simulink model "Sistema_completo"  (R2020b)
settings: Solver=FixedStepAuto  StartTime=0.0  StopTime=inf  FixedStep=0.01  RelTol=1e-3  EnableMultiTasking=on
values from neighbouring files (symbols this model uses):
  a_c_max = 1    [Parametros_y_Simulacion.m]
  a_i_max = 1    [Parametros_y_Simulacion.m]
  b_cx = 1000.0    (= 1000)    [Parametros_y_Simulacion.m]
  b_cy = 500.0    (= 500)    [Parametros_y_Simulacion.m]
  b_eqc = b_eq * r_t^2 / R_r^2    (= 27000)    [Parametros_y_Simulacion.m]
  b_eqi = b_eq2 * r_ti^2 / R_d^2    (= 28800)    [Parametros_y_Simulacion.m]
  b_w = 30000.0    (= 30000)    [Parametros_y_Simulacion.m]
  g = 9.81    [Parametros_y_Simulacion.m]
  H_colmn = [34,34, 19,19, 35,30, 35,30, 23]    [Parametros_y_Simulacion.m]
  H_contenedor = 2.5    [Parametros_y_Simulacion.m]
  H_seguridad = 5    [Parametros_y_Simulacion.m]
  K_cy = 1.3e6    (= 1300000)    [Parametros_y_Simulacion.m]
  K_w = 1800000.0    (= 1800000)    [Parametros_y_Simulacion.m]
  L_colmn = [5,10,15, 20,25, 30,35, 40,45]    [Parametros_y_Simulacion.m]
  l_t0 = y_t0 - H_contenedor - H_seguridad -(m_spreader * g) / K_w    (= 37.41825)    [Parametros_y_Simulacion.m]
  m_carga = 48000.0    (= 48000)    [Parametros_y_Simulacion.m]
  m_eqc = m_c + (J_r + J_m * r_t^2) / (R_r^2)    (= 59008)    [Parametros_y_Simulacion.m]
  m_eqi = (J_d + J_mi * r_ti^2) / R_d^2    (= 48014.2222222)    [Parametros_y_Simulacion.m]
  m_spreader = 15000.0    (= 15000)    [Parametros_y_Simulacion.m]
  omega_c_mod = 1000    [Parametros_y_Simulacion.m]
  omega_i_mod = 1000    [Parametros_y_Simulacion.m]
  R_d = 0.75    [Parametros_y_Simulacion.m]
  R_r = 0.5    [Parametros_y_Simulacion.m]
  r_t = 15.0    (= 15)    [Parametros_y_Simulacion.m]
  r_ti = 30.0    (= 30)    [Parametros_y_Simulacion.m]
  v_c_max = 4    [Parametros_y_Simulacion.m]
  x_t0 = -20    [Parametros_y_Simulacion.m]
  y_t0 = 45    [Parametros_y_Simulacion.m]
undefined symbols (not defined in the file or in its folder): B_ac, B_ai, H, K_db, K_pb, K_sac, K_sai, K_siac, K_siai, L, lh
libraries: aerolibanimutils x1
settings Model: Creator=Facundo  LastModifiedBy=tinsu
settings DataIOCC: LimitDataPoints=on  ReturnWorkspaceOutputs=off
settings OptimizationCC: ZeroExternalMemoryAtStartup=off  ZeroInternalMemoryAtStartup=off  LifeSpan=inf
settings DebuggingCC: SFUnexpectedBacktrackingDiag=warning  SFNoUnconditionalDefaultTransitionDiag=warning  SFExecutionAtInitializationDiag=none  ArithmeticOperatorsInVariantConditions=warning
settings HardwareCC: ProdBitPerSizeT=32  ProdBitPerPtrDiffT=32  ProdWordSize=32  ProdHWDeviceType=Specified
settings ModelReferenceCC: PropagateSignalLabelsOutOfModel=off
settings SFSimCC: SimUseLocalCustomCode=off  CustomCodeUndefinedFunction=UseInterfaceOnly  SimTargetLang=C++
settings RTWCC: RTWUseLocalCustomCode=off  TargetLang=C++
settings CodeAppCC: StateflowObjectComments=on
settings GRTTargetCC: TargetLangStandard=C89/C90 (ANSI)  CodeInterfacePackaging=C++ class  RTWCAPISignals=on
settings ConfigComp: CovMetricSettings=dw  CovSaveCumulativeToWorkspaceVar=on  CovSaveSingleToWorkspaceVar=on  CovExternalEMLEnable=off

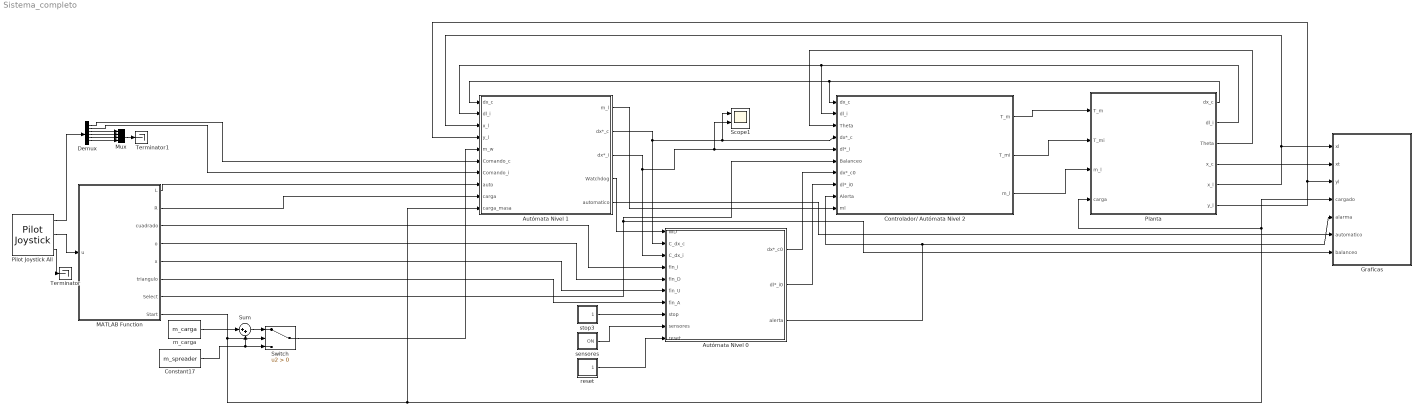
== system Sistema_completo ==
  " Planta" : Subsystem
  Autómata Nivel 0 : Subsystem
  Autómata Nivel 1 : Subsystem
  Constant17 : Constant  Value=m_spreader
  Controlador/ Autómata Nivel 2 : Subsystem
  Demux : Demux  Outputs=6
  Graficas : Stateflow chart  TreatAsAtomicUnit=on
  MATLAB Function : MATLAB Function  TreatAsAtomicUnit=on
  Mux : Mux
  Pilot Joystick All : aerolibanimutils/Pilot Joystick  JoystickID=Joystick1  OutputConfiguration=AllOutputs  SampleTime=0.01
  Scope1 : Scope  NumInputPorts=2
  Sum : Sum  Inputs=|++
  Switch : Switch  Criteria=u2 > Threshold
  Terminator : Terminator
  Terminator1 : Terminator
  m_carga : Constant  Value=m_carga
  reset : Subsystem
      settings: OpenFcn=|
      | blockname1=[gcb '/ControlValue/'];
      | blockname2=[gcb '/'];
      | 
      | h1=get_param(blockname1,'handle');
      | h2=get_param(blockname2,'handle');
      | ONOFF=str2num(get_param(h1,'Value'));
      | 
      | if ONOFF== 1
      |     %Turn off
      |     set_param(h1,'Value','-1')
      |     set_param(h2,'BackgroundColor','blue')
      |     set_param([gcb '/ON'],'Name','OFF')
      | else
      |     %Turn on
      |     set_param(h1,'Value','1')
      |     set_param(h2,'BackgroundColor','red')
      |     set_param([gcb '/OFF'],'Name','ON')
      | end
  sensores : Subsystem
      settings: OpenFcn=|
      | blockname1=[gcb '/ControlValue/'];
      | blockname2=[gcb '/'];
      | 
      | h1=get_param(blockname1,'handle');
      | h2=get_param(blockname2,'handle');
      | ONOFF=str2num(get_param(h1,'Value'));
      | 
      | if ONOFF== 1
      |     %Turn off
      |     set_param(h1,'Value','-1')
      |     set_param(h2,'BackgroundColor','blue')
      |     set_param([gcb '/ON'],'Name','OFF')
      | else
      |     %Turn on
      |     set_param(h1,'Value','1')
      |     set_param(h2,'BackgroundColor','red')
      |     set_param([gcb '/OFF'],'Name','ON')
      | end
  stop3 : Subsystem
      settings: OpenFcn=|
      | blockname1=[gcb '/ControlValue/'];
      | blockname2=[gcb '/'];
      | 
      | h1=get_param(blockname1,'handle');
      | h2=get_param(blockname2,'handle');
      | ONOFF=str2num(get_param(h1,'Value'));
      | 
      | if ONOFF== 1
      |     %Turn off
      |     set_param(h1,'Value','-1')
      |     set_param(h2,'BackgroundColor','blue')
      |     set_param([gcb '/ON'],'Name','OFF')
      | else
      |     %Turn on
      |     set_param(h1,'Value','1')
      |     set_param(h2,'BackgroundColor','red')
      |     set_param([gcb '/OFF'],'Name','ON')
      | end
  wires:
  " Planta"/4(x_c) -> Graficas/2(xt)
  MATLAB Function/7(Select) -> Graficas/7(balanceo), Controlador/ Autómata Nivel 2/6(Balanceo)
  Autómata Nivel 0/3(alerta) -> Controlador/ Autómata Nivel 2/9(Alerta), Graficas/5(alarma)
  MATLAB Function/6(triangulo) -> Autómata Nivel 0/7(fin_A)
  Demux/4 -> Mux/2
  Constant17/1 -> Sum/2, Switch/3
  m_carga/1 -> Sum/1
  MATLAB Function/3(cuadrado) -> Autómata Nivel 0/4(fin_I)
  Demux/5 -> Mux/3
  Sum/1 -> Switch/1
  Switch/1 -> Autómata Nivel 1/5(m_w)
  Pilot Joystick All/1 -> Demux/1
  MATLAB Function/4(o) -> Autómata Nivel 0/5(fin_D)
  MATLAB Function/5(x) -> Autómata Nivel 0/6(fin_U)
  MATLAB Function/1(L) -> Autómata Nivel 1/8(auto)
  MATLAB Function/2(R) -> Autómata Nivel 1/9(carga)
  Mux/1 -> Terminator1/1
  Pilot Joystick All/2 -> MATLAB Function/1(u)
  Demux/3 -> Mux/1
  Demux/6 -> Mux/4
  Pilot Joystick All/3 -> Terminator/1
  " Planta"/5(x_l) -> Autómata Nivel 1/3(x_l), Graficas/1(xl)
  " Planta"/6(y_l) -> Autómata Nivel 1/4(y_l), Graficas/3(yl)
  stop3/1(OFF) -> Autómata Nivel 0/8(stop)
  sensores/1(ON) -> Autómata Nivel 0/9(sensores)
  reset/1(OFF) -> Autómata Nivel 0/10(reset)
  Controlador/ Autómata Nivel 2/1(T_m) -> " Planta"/1(T_m)
  Controlador/ Autómata Nivel 2/2(T_mi) -> " Planta"/2(T_mi)
  Controlador/ Autómata Nivel 2/3(m_l) -> " Planta"/3(m_l)
  " Planta"/3(Theta) -> Controlador/ Autómata Nivel 2/3(Theta)
  " Planta"/1(dx_c) -> Controlador/ Autómata Nivel 2/1(dx_c), Autómata Nivel 1/1(dx_c)
  " Planta"/2(dl_i) -> Controlador/ Autómata Nivel 2/2(dl_i), Autómata Nivel 1/2(dl_i)
  Autómata Nivel 0/1(dx*_c0) -> Controlador/ Autómata Nivel 2/7(dx*_c0)
  Autómata Nivel 0/2(dl*_i0) -> Controlador/ Autómata Nivel 2/8(dl*_i0)
  Autómata Nivel 1/1(m_l) -> Controlador/ Autómata Nivel 2/10(ml)
  Autómata Nivel 1/2(dx*_c) -> Scope1/1, Controlador/ Autómata Nivel 2/4(dx*_c), Autómata Nivel 0/2(C_dx_c)
  Autómata Nivel 1/3(dx*_i) -> Scope1/2, Controlador/ Autómata Nivel 2/5(dl*_i), Autómata Nivel 0/3(C_dx_i)
  Autómata Nivel 1/4(Watchdog) -> Autómata Nivel 0/1(WD)
  Autómata Nivel 1/5(automatico) -> Graficas/6(automatico)
  Demux/1 -> Autómata Nivel 1/6(Comando_c)
  Demux/2 -> Autómata Nivel 1/7(Comando_i)
  MATLAB Function/8(Start) -> Switch/2, Autómata Nivel 1/10(carga_masa), " Planta"/4(carga), Graficas/4(cargado)

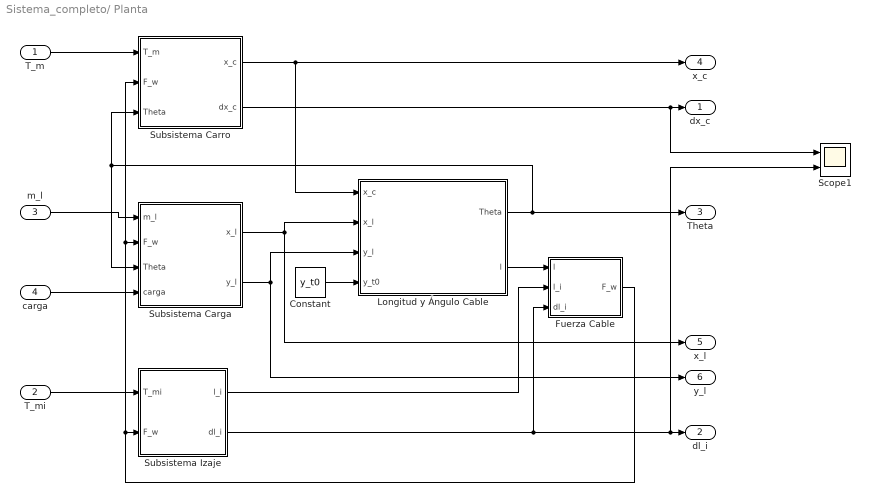
== system Sistema_completo/ Planta ==
  T_m : Inport
  T_mi : Inport  Port=2
  m_l : Inport  Port=3
  carga : Inport  Port=4
  " Fuerza Cable" : Subsystem
  Constant : Constant  Value=y_t0
  Longitud y Ángulo Cable : MATLAB Function  TreatAsAtomicUnit=on
  Scope1 : Scope  NumInputPorts=2
  Subsistema Carga : Subsystem
  Subsistema Carro : Subsystem
  Subsistema Izaje : Subsystem
  dx_c : Outport  VectorParamsAs1DForOutWhenUnconnected=off
  dl_i : Outport  Port=2  VectorParamsAs1DForOutWhenUnconnected=off
  Theta : Outport  Port=3  VectorParamsAs1DForOutWhenUnconnected=off
  x_c : Outport  Port=4  VectorParamsAs1DForOutWhenUnconnected=off
  x_l : Outport  Port=5  VectorParamsAs1DForOutWhenUnconnected=off
  y_l : Outport  Port=6  VectorParamsAs1DForOutWhenUnconnected=off
  wires:
  Constant/1 -> Longitud y Ángulo Cable/4(y_t0)
  Subsistema Carro/1(x_c) -> Longitud y Ángulo Cable/1(x_c), x_c/1
  Subsistema Carga/1(x_l) -> Longitud y Ángulo Cable/2(x_l), x_l/1
  Subsistema Carga/2(y_l) -> Longitud y Ángulo Cable/3(y_l), y_l/1
  Longitud y Ángulo Cable/2(l) -> " Fuerza Cable"/1(l)
  Subsistema Izaje/1(l_i) -> " Fuerza Cable"/2(l_i)
  Subsistema Izaje/2(dl_i) -> " Fuerza Cable"/3(dl_i), Scope1/2, dl_i/1
  " Fuerza Cable"/1(F_w) -> Subsistema Carga/2(F_w), Subsistema Carro/2(F_w), Subsistema Izaje/2(F_w)
  Longitud y Ángulo Cable/1(Theta) -> Theta/1, Subsistema Carga/3(Theta), Subsistema Carro/3(Theta)
  T_m/1 -> Subsistema Carro/1(T_m)
  m_l/1 -> Subsistema Carga/1(m_l)
  T_mi/1 -> Subsistema Izaje/1(T_mi)
  Subsistema Carro/2(dx_c) -> Scope1/1, dx_c/1
  carga/1 -> Subsistema Carga/4(carga)

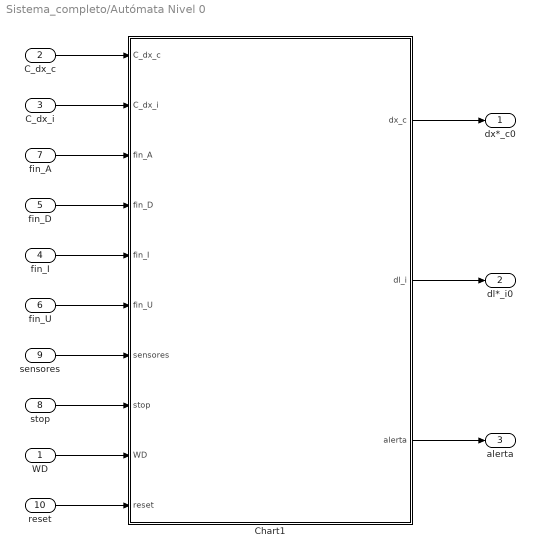
== system Sistema_completo/Autómata Nivel 0 ==
  WD : Inport
  C_dx_c : Inport  Port=2
  C_dx_i : Inport  Port=3
  fin_I : Inport  Port=4
  fin_D : Inport  Port=5
  fin_U : Inport  Port=6
  fin_A : Inport  Port=7
  stop : Inport  Port=8
  sensores : Inport  Port=9
  reset : Inport  Port=10
  Chart1 : Stateflow chart  TreatAsAtomicUnit=on
  dx*_c0 : Outport
  dl*_i0 : Outport  Port=2
  alerta : Outport  Port=3
  wires:
  stop/1 -> Chart1/8(stop)
  C_dx_i/1 -> Chart1/2(C_dx_i)
  fin_D/1 -> Chart1/4(fin_D)
  fin_A/1 -> Chart1/3(fin_A)
  fin_U/1 -> Chart1/6(fin_U)
  sensores/1 -> Chart1/7(sensores)
  fin_I/1 -> Chart1/5(fin_I)
  C_dx_c/1 -> Chart1/1(C_dx_c)
  WD/1 -> Chart1/9(WD)
  Chart1/3(alerta) -> alerta/1
  Chart1/2(dl_i) -> dl*_i0/1
  Chart1/1(dx_c) -> dx*_c0/1
  reset/1 -> Chart1/10(reset)

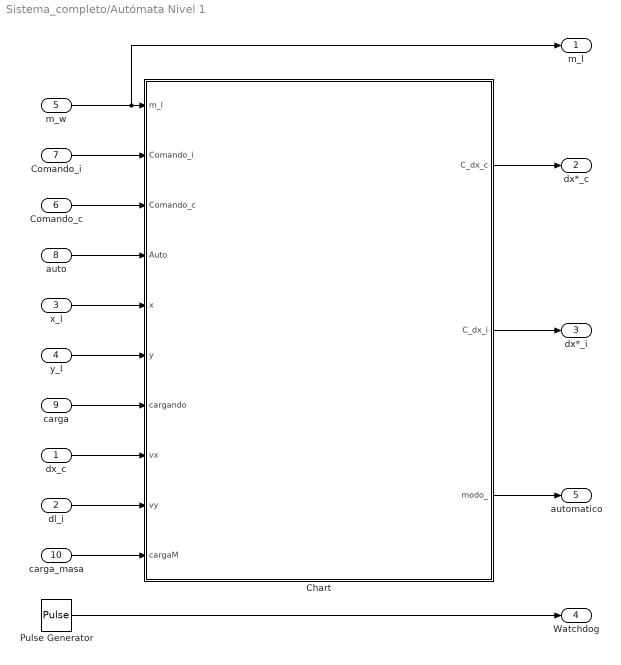
== system Sistema_completo/Autómata Nivel 1 ==
  dx_c : Inport
  dl_i : Inport  Port=2
  x_l : Inport  Port=3
  y_l : Inport  Port=4
  m_w : Inport  Port=5
  Comando_c : Inport  Port=6
  Comando_i : Inport  Port=7
  auto : Inport  Port=8
  carga : Inport  Port=9
  carga_masa : Inport  Port=10
  Chart : Stateflow chart  TreatAsAtomicUnit=on
  Pulse Generator : DiscretePulseGenerator  PulseType=Time based  Period=0.2  PulseWidth=50  PhaseDelay=0.1
  m_l : Outport  VectorParamsAs1DForOutWhenUnconnected=off
  dx*_c : Outport  Port=2  VectorParamsAs1DForOutWhenUnconnected=off
  dx*_i : Outport  Port=3  VectorParamsAs1DForOutWhenUnconnected=off
  Watchdog : Outport  Port=4
  automatico : Outport  Port=5
  wires:
  Chart/1(C_dx_c) -> dx*_c/1
  y_l/1 -> Chart/6(y)
  Comando_i/1 -> Chart/2(Comando_i)
  m_w/1 -> m_l/1, Chart/1(m_l)
  Chart/2(C_dx_i) -> dx*_i/1
  auto/1 -> Chart/4(Auto)
  x_l/1 -> Chart/5(x)
  carga/1 -> Chart/7(cargando)
  Comando_c/1 -> Chart/3(Comando_c)
  Pulse Generator/1 -> Watchdog/1
  dx_c/1 -> Chart/8(vx)
  dl_i/1 -> Chart/9(vy)
  Chart/3(modo_) -> automatico/1
  carga_masa/1 -> Chart/10(cargaM)

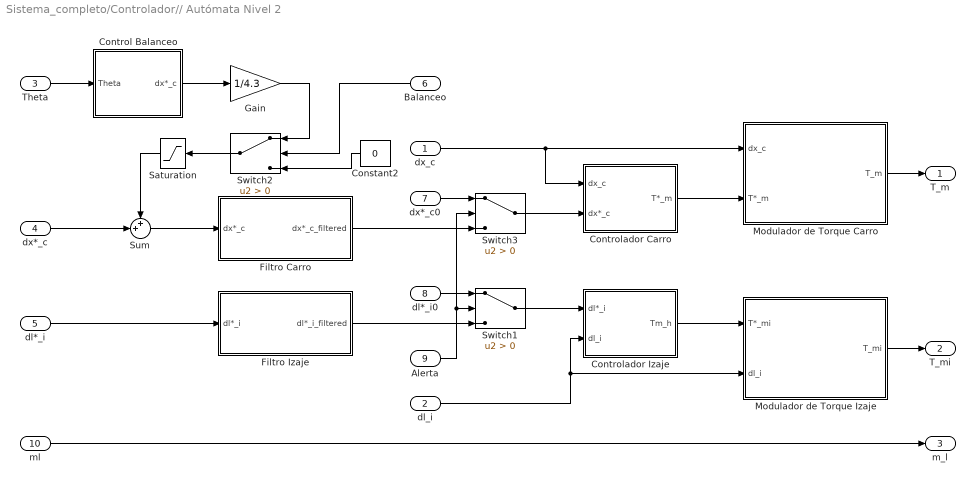
== system Sistema_completo/Controlador// Autómata Nivel 2 ==
  dx_c : Inport
  dl_i : Inport  Port=2
  Theta : Inport  Port=3
  dx*_c : Inport  Port=4
  dl*_i : Inport  Port=5
  Balanceo : Inport  Port=6
  dx*_c0 : Inport  Port=7
  dl*_i0 : Inport  Port=8
  Alerta : Inport  Port=9
  ml : Inport  Port=10
  Constant2 : Constant  Value=0
  Control Balanceo : Subsystem
  Controlador Carro : Subsystem
  Controlador Izaje : Subsystem
  Filtro Carro : Subsystem
  Filtro Izaje : Subsystem
  Gain : Gain  Gain=1/4.3
  Modulador de Torque Carro : Subsystem
  Modulador de Torque Izaje : Subsystem
  "Saturation " : Saturate  UpperLimit=5  LowerLimit=-5
  Sum : Sum  Inputs=++|
  Switch1 : Switch  Criteria=u2 > Threshold
  Switch2 : Switch  Criteria=u2 > Threshold
  Switch3 : Switch  Criteria=u2 > Threshold
  T_m : Outport  VectorParamsAs1DForOutWhenUnconnected=off
  T_mi : Outport  Port=2  VectorParamsAs1DForOutWhenUnconnected=off
  m_l : Outport  Port=3  VectorParamsAs1DForOutWhenUnconnected=off
  wires:
  ml/1 -> m_l/1
  Theta/1 -> Control Balanceo/1(Theta)
  Gain/1 -> Switch2/1
  Control Balanceo/1(dx*_c) -> Gain/1
  dl_i/1 -> Controlador Izaje/2(dl_i), Modulador de Torque Izaje/2(dl_i)
  Switch1/1 -> Controlador Izaje/1(dl*_i)
  Switch3/1 -> Controlador Carro/2(dx*_c)
  dl*_i0/1 -> Switch1/1
  Alerta/1 -> Switch3/2, Switch1/2
  dx*_c0/1 -> Switch3/1
  "Saturation "/1 -> Sum/1
  Switch2/1 -> "Saturation "/1
  Constant2/1 -> Switch2/3
  Balanceo/1 -> Switch2/2
  dx*_c/1 -> Sum/2
  dx_c/1 -> Controlador Carro/1(dx_c), Modulador de Torque Carro/1(dx_c)
  Modulador de Torque Carro/1(T_m) -> T_m/1
  Modulador de Torque Izaje/1(T_mi) -> T_mi/1
  Controlador Carro/1(T*_m) -> Modulador de Torque Carro/2(T*_m)
  Controlador Izaje/1(Tm_h) -> Modulador de Torque Izaje/1(T*_mi)
  Sum/1 -> Filtro Carro/1(dx*_c)
  Filtro Carro/1(dx*_c_filtered) -> Switch3/3
  dl*_i/1 -> Filtro Izaje/1(dl*_i)
  Filtro Izaje/1(dl*_i_filtered) -> Switch1/3

== system Sistema_completo/reset ==
  ControlValue : Constant  Value=-1
  Off : Constant  Value=0
  On : Constant
  Switch : Switch
  OFF : Outport  VectorParamsAs1DForOutWhenUnconnected=off
  wires:
  On/1 -> Switch/1
  Off/1 -> Switch/3
  ControlValue/1 -> Switch/2
  Switch/1 -> OFF/1

== system Sistema_completo/sensores ==
  ControlValue : Constant
  Off : Constant  Value=0
  On : Constant
  Switch : Switch
  ON : Outport  VectorParamsAs1DForOutWhenUnconnected=off
  wires:
  On/1 -> Switch/1
  Off/1 -> Switch/3
  ControlValue/1 -> Switch/2
  Switch/1 -> ON/1

== system Sistema_completo/stop3 ==
  ControlValue : Constant  Value=-1
  Off : Constant  Value=0
  On : Constant
  Switch : Switch
  OFF : Outport  VectorParamsAs1DForOutWhenUnconnected=off
  wires:
  On/1 -> Switch/1
  Off/1 -> Switch/3
  ControlValue/1 -> Switch/2
  Switch/1 -> OFF/1

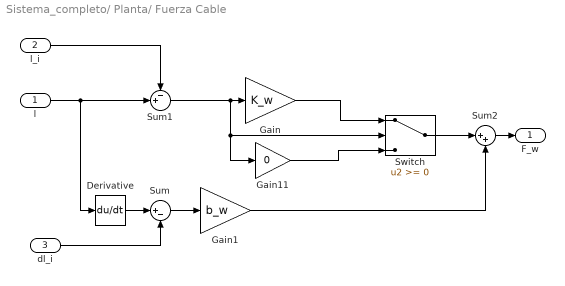
== system Sistema_completo/ Planta/ Fuerza Cable ==
  l : Inport
  l_i : Inport  Port=2
  dl_i : Inport  Port=3
  Derivative : Derivative
  Gain : Gain  Gain=K_w
  Gain1 : Gain  Gain=b_w
  Gain11 : Gain  Gain=0
  Sum : Sum  Inputs=|+-
  Sum1 : Sum  Inputs=-+|
  Sum2 : Sum  Inputs=|++
  Switch : Switch
  F_w : Outport  VectorParamsAs1DForOutWhenUnconnected=off
  wires:
  dl_i/1 -> Sum/2
  l_i/1 -> Sum1/1
  Derivative/1 -> Sum/1
  Sum1/1 -> Switch/2, Gain11/1, Gain/1
  Sum/1 -> Gain1/1
  l/1 -> Derivative/1, Sum1/2
  Sum2/1 -> F_w/1
  Gain1/1 -> Sum2/2
  Switch/1 -> Sum2/1
  Gain11/1 -> Switch/3
  Gain/1 -> Switch/1

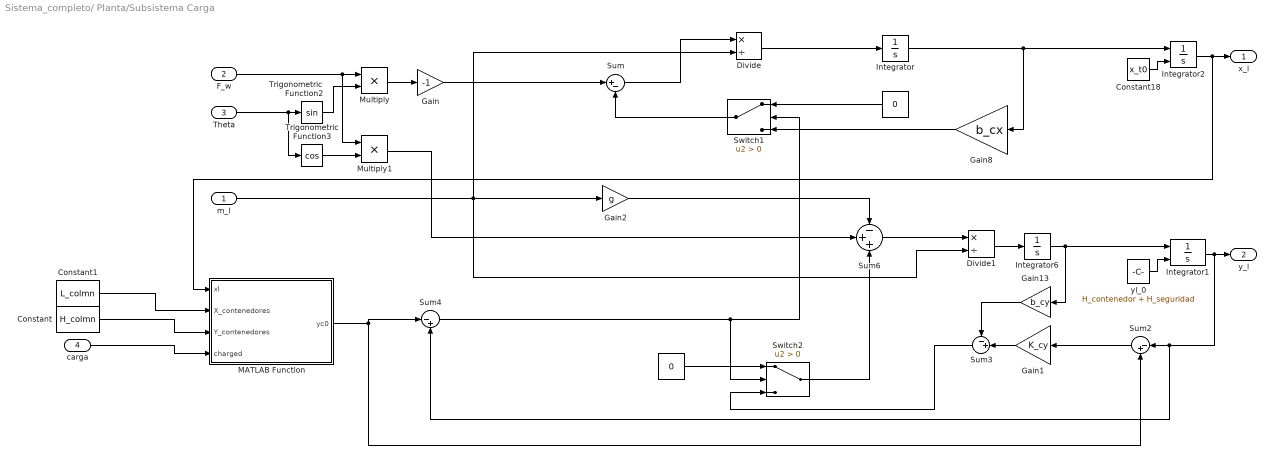
== system Sistema_completo/ Planta/Subsistema Carga ==
  m_l : Inport
  F_w : Inport  Port=2
  Theta : Inport  Port=3
  carga : Inport  Port=4
  " " : Constant  Value=0
  "   " : Constant  Value=0
  Constant : Constant  Value=H_colmn
  Constant1 : Constant  Value=L_colmn
  Constant18 : Constant  Value=x_t0
  Divide : Product  Inputs=*/
  Divide1 : Product  Inputs=*/
  Gain : Gain  Gain=-1
  Gain1 : Gain  Gain=K_cy
  Gain13 : Gain  Gain=b_cy
  Gain2 : Gain  Gain=g
  Gain8 : Gain  Gain=b_cx
  Integrator : Integrator
  Integrator1 : Integrator  InitialConditionSource=external
  Integrator2 : Integrator  InitialConditionSource=external
  Integrator6 : Integrator
  MATLAB Function : MATLAB Function  TreatAsAtomicUnit=on
  Multiply : Product
  Multiply1 : Product
  Sum : Sum  Inputs=|+-
  Sum2 : Sum  Inputs=|-+
  Sum3 : Sum  Inputs=-+|
  Sum4 : Sum  Inputs=|-+
  Sum6 : Sum  Inputs=-++
  Switch1 : Switch  Criteria=u2 > Threshold
  Switch2 : Switch  Criteria=u2 > Threshold
  Trigonometric Function2 : Trigonometry
  Trigonometric Function3 : Trigonometry  Operator=cos
  yl_0 : Constant  Value=H_contenedor + H_seguridad
  x_l : Outport  VectorParamsAs1DForOutWhenUnconnected=off
  y_l : Outport  Port=2  VectorParamsAs1DForOutWhenUnconnected=off
  wires:
  Divide1/1 -> Integrator6/1
  Integrator2/1 -> MATLAB Function/1(xl), x_l/1
  Integrator6/1 -> Gain13/1, Integrator1/1
  Gain/1 -> Sum/1
  F_w/1 -> Multiply1/1, Multiply/1
  Trigonometric Function2/1 -> Multiply/2
  Trigonometric Function3/1 -> Multiply1/2
  m_l/1 -> Divide1/2, Divide/2, Gain2/1
  Divide/1 -> Integrator/1
  Constant18/1 -> Integrator2/2
  Integrator/1 -> Gain8/1, Integrator2/1
  Integrator1/1 -> Sum4/2, Sum2/1, y_l/1
  yl_0/1 -> Integrator1/2
  Theta/1 -> Trigonometric Function3/1, Trigonometric Function2/1
  Multiply/1 -> Gain/1
  Multiply1/1 -> Sum6/2
  Gain8/1 -> Switch1/3
  Switch1/1 -> Sum/2
  Sum/1 -> Divide/1
  " "/1 -> Switch1/1
  Sum2/1 -> Gain1/1
  Gain1/1 -> Sum3/2
  Gain13/1 -> Sum3/1
  Sum3/1 -> Switch2/3
  "   "/1 -> Switch2/1
  Switch2/1 -> Sum6/3
  MATLAB Function/1(yc0) -> Sum4/1, Sum2/2
  Sum4/1 -> Switch2/2, Switch1/2
  Gain2/1 -> Sum6/1
  Sum6/1 -> Divide1/1
  Constant/1 -> MATLAB Function/3(Y_contenedores)
  carga/1 -> MATLAB Function/4(charged)
  Constant1/1 -> MATLAB Function/2(X_contenedores)

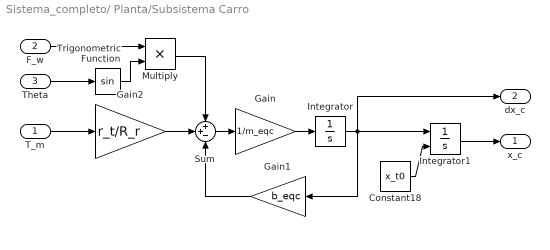
== system Sistema_completo/ Planta/Subsistema Carro ==
  T_m : Inport
  F_w : Inport  Port=2
  Theta : Inport  Port=3
  Constant18 : Constant  Value=x_t0
  Gain : Gain  Gain=1/m_eqc
  Gain1 : Gain  Gain=b_eqc
  Gain2 : Gain  Gain=r_t/R_r
  Integrator : Integrator
  Integrator1 : Integrator  InitialConditionSource=external
  Multiply : Product
  Sum : Sum  Inputs=++-
  Trigonometric Function : Trigonometry
  x_c : Outport  VectorParamsAs1DForOutWhenUnconnected=off
  dx_c : Outport  Port=2  VectorParamsAs1DForOutWhenUnconnected=off
  wires:
  Gain/1 -> Integrator/1
  Sum/1 -> Gain/1
  Gain1/1 -> Sum/3
  T_m/1 -> Gain2/1
  Trigonometric Function/1 -> Multiply/2
  Theta/1 -> Trigonometric Function/1
  F_w/1 -> Multiply/1
  Integrator/1 -> Integrator1/1, Gain1/1, dx_c/1
  Constant18/1 -> Integrator1/2
  Integrator1/1 -> x_c/1
  Gain2/1 -> Sum/2
  Multiply/1 -> Sum/1

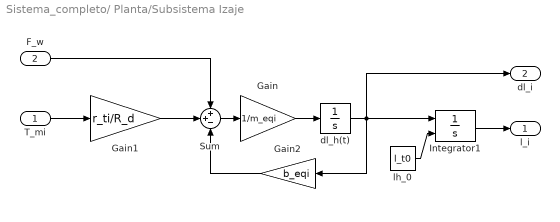
== system Sistema_completo/ Planta/Subsistema Izaje ==
  T_mi : Inport
  F_w : Inport  Port=2
  Gain : Gain  Gain=1/m_eqi
  Gain1 : Gain  Gain=r_ti/R_d
  Gain2 : Gain  Gain=b_eqi
  Integrator1 : Integrator  InitialConditionSource=external
  Sum : Sum  Inputs=++-
  dl_h(t) : Integrator
  lh_0 : Constant  Value=l_t0
  l_i : Outport  VectorParamsAs1DForOutWhenUnconnected=off
  dl_i : Outport  Port=2  VectorParamsAs1DForOutWhenUnconnected=off
  wires:
  F_w/1 -> Sum/1
  T_mi/1 -> Gain1/1
  Integrator1/1 -> l_i/1
  Gain1/1 -> Sum/2
  Gain2/1 -> Sum/3
  Sum/1 -> Gain/1
  dl_h(t)/1 -> dl_i/1, Integrator1/1, Gain2/1
  lh_0/1 -> Integrator1/2
  Gain/1 -> dl_h(t)/1

== system Sistema_completo/Controlador// Autómata Nivel 2/Control Balanceo ==
  Theta : Inport
  Derivative1 : Derivative
  Gain : Gain  Gain=-1
  Gain4 : Gain  Gain=K_pb(abs(lh))
  Gain5 : Gain  Gain=K_db(abs(lh))
  Sum1 : Sum  Inputs=+|+
  dx*_c : Outport  VectorParamsAs1DForOutWhenUnconnected=off
  wires:
  Gain/1 -> Gain4/1, Derivative1/1
  Gain4/1 -> Sum1/1
  Gain5/1 -> Sum1/2
  Sum1/1 -> dx*_c/1
  Theta/1 -> Gain/1
  Derivative1/1 -> Gain5/1

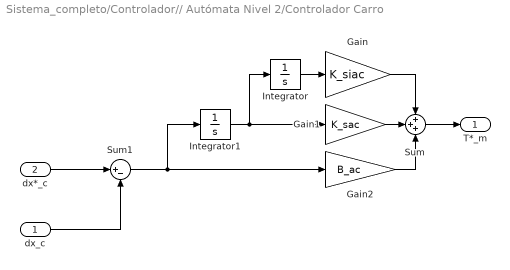
== system Sistema_completo/Controlador// Autómata Nivel 2/Controlador Carro ==
  dx_c : Inport
  dx*_c : Inport  Port=2
  Gain : Gain  Gain=K_siac
  Gain1 : Gain  Gain=K_sac
  Gain2 : Gain  Gain=B_ac
  Integrator : Integrator
  Integrator1 : Integrator
  Sum : Sum  Inputs=+++
  Sum1 : Sum  Inputs=|+-
  T*_m : Outport  VectorParamsAs1DForOutWhenUnconnected=off
  wires:
  Gain1/1 -> Sum/2
  Integrator/1 -> Gain/1
  Integrator1/1 -> Gain1/1, Integrator/1
  Sum/1 -> T*_m/1
  Gain/1 -> Sum/1
  Gain2/1 -> Sum/3
  dx*_c/1 -> Sum1/1
  dx_c/1 -> Sum1/2
  Sum1/1 -> Gain2/1, Integrator1/1

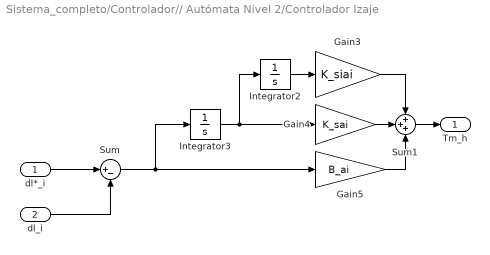
== system Sistema_completo/Controlador// Autómata Nivel 2/Controlador Izaje ==
  dl*_i : Inport
  dl_i : Inport  Port=2
  Gain3 : Gain  Gain=K_siai
  Gain4 : Gain  Gain=K_sai
  Gain5 : Gain  Gain=B_ai
  Integrator2 : Integrator
  Integrator3 : Integrator
  Sum : Sum  Inputs=|+-
  Sum1 : Sum  Inputs=+++
  Tm_h : Outport  VectorParamsAs1DForOutWhenUnconnected=off
  wires:
  Gain4/1 -> Sum1/2
  Integrator2/1 -> Gain3/1
  Integrator3/1 -> Gain4/1, Integrator2/1
  Sum1/1 -> Tm_h/1
  Gain3/1 -> Sum1/1
  Gain5/1 -> Sum1/3
  Sum/1 -> Integrator3/1, Gain5/1
  dl*_i/1 -> Sum/1
  dl_i/1 -> Sum/2

== system Sistema_completo/Controlador// Autómata Nivel 2/Filtro Carro ==
  dx*_c : Inport
  2 : Gain  Gain=4
  "Rate Limiter " : RateLimiter  RisingSlewLimit=a_c_max  FallingSlewLimit=-a_c_max
  Sum3 : Sum  Inputs=|+-
  dl_h(t)2 : Integrator
  dx*_c_filtered : Outport  VectorParamsAs1DForOutWhenUnconnected=off
  wires:
  Sum3/1 -> dl_h(t)2/1
  2/1 -> dx*_c_filtered/1, Sum3/2
  "Rate Limiter "/1 -> Sum3/1
  dl_h(t)2/1 -> 2/1
  dx*_c/1 -> "Rate Limiter "/1

== system Sistema_completo/Controlador// Autómata Nivel 2/Filtro Izaje ==
  dl*_i : Inport
  1 : Gain  Gain=10
  Rate Limiter : RateLimiter  RisingSlewLimit=a_i_max  FallingSlewLimit=-a_i_max
  Sum4 : Sum  Inputs=|+-
  dl_h(t)1 : Integrator
  dl*_i_filtered : Outport  VectorParamsAs1DForOutWhenUnconnected=off
  wires:
  dl_h(t)1/1 -> 1/1
  1/1 -> dl*_i_filtered/1, Sum4/2
  Sum4/1 -> dl_h(t)1/1
  dl*_i/1 -> Rate Limiter/1
  Rate Limiter/1 -> Sum4/1

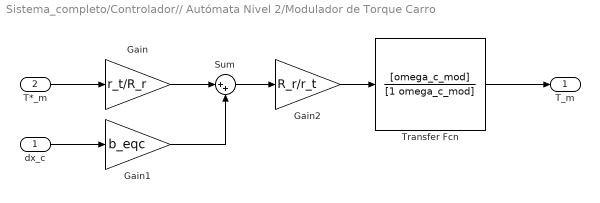
== system Sistema_completo/Controlador// Autómata Nivel 2/Modulador de Torque Carro ==
  dx_c : Inport
  T*_m : Inport  Port=2
  Gain : Gain  Gain=r_t/R_r
  Gain1 : Gain  Gain=b_eqc
  Gain2 : Gain  Gain=R_r/r_t
  Sum : Sum  Inputs=|++
  Transfer Fcn : TransferFcn  Numerator=[omega_c_mod]  Denominator=[1 omega_c_mod]
  T_m : Outport  VectorParamsAs1DForOutWhenUnconnected=off
  wires:
  Transfer Fcn/1 -> T_m/1
  dx_c/1 -> Gain1/1
  Gain/1 -> Sum/1
  Gain2/1 -> Transfer Fcn/1
  Sum/1 -> Gain2/1
  Gain1/1 -> Sum/2
  T*_m/1 -> Gain/1

== system Sistema_completo/Controlador// Autómata Nivel 2/Modulador de Torque Izaje ==
  T*_mi : Inport
  dl_i : Inport  Port=2
  Gain : Gain  Gain=r_ti/R_d
  Gain1 : Gain  Gain=b_eqi
  Gain2 : Gain  Gain=R_d/r_ti
  Sum : Sum  Inputs=|++
  Transfer Fcn : TransferFcn  Numerator=[omega_i_mod]  Denominator=[1 omega_i_mod]
  T_mi : Outport  VectorParamsAs1DForOutWhenUnconnected=off
  wires:
  Transfer Fcn/1 -> T_mi/1
  Gain2/1 -> Transfer Fcn/1
  dl_i/1 -> Gain1/1
  Gain1/1 -> Sum/2
  Gain/1 -> Sum/1
  Sum/1 -> Gain2/1
  T*_mi/1 -> Gain/1

== stateflow chart Sistema_completo/Autómata Nivel 1/Chart ==
  state MOVIMIENTO [parallel]
    during:
    v_i_max = vMaxIzaje(m_l);
    settings: executionOrder=2
    state MANUAL
      entry:
      modo_=0;
      state CARRO [parallel]
        settings: executionOrder=1
        state NORMAL
          during:
          C_dx_c = Comando_c * v_c_max;
        (default) -> MOVIMIENTO.MANUAL.CARRO.NORMAL
      state IZAJE [parallel]
        settings: executionOrder=2
        state NORMAL
          during:
          C_dx_i = Comando_i * v_i_max;
        (default) -> MOVIMIENTO.MANUAL.IZAJE.NORMAL
    state AUTOMATICO
      entry:
      modo_=1;
      state CARRO [parallel]
        settings: executionOrder=1
        state INICIO
        state RETROCESO
          during:
          C_dx_c = -v_c_max;
        state AVANCE
          during:
          C_dx_c = v_c_max;
        state DETENCION
          during:
          C_dx_c = 0;
        (default) -> MOVIMIENTO.AUTOMATICO.CARRO.INICIO
        MOVIMIENTO.AUTOMATICO.CARRO.INICIO -> AVANCE [order 1] : [(etapa == 1 || etapa == 2) && cargando]
        MOVIMIENTO.AUTOMATICO.CARRO.INICIO -> RETROCESO [order 2] : [(etapa == 4 || etapa == 3) && ~cargando]
        MOVIMIENTO.AUTOMATICO.CARRO.INICIO -> DETENCION [order 3] : [(etapa == 4 || etapa == 3) && cargando || (etapa == 1) && ~cargando]
        RETROCESO -> DETENCION : [etapa == 2]
        AVANCE -> DETENCION : [etapa == 3]
      state IZAJE [parallel]
        settings: executionOrder=2
        state ASCENSO_C
          during:
          C_dx_i = -v_i_max;
        state DETENCION_C
          during:
          C_dx_i = 0;
        state DESCENSO_C
          during:
          C_dx_i = v_i_max;
        state INICIO
          entry:
          C_dx_i = 0;
        state DETENCION_D
          during:
          C_dx_i = 0;
        state DESCENSO_D
          during:
          C_dx_i = v_i_max;
        state ASCENSO_D
          during:
          C_dx_i = -v_i_max;
        ASCENSO_C -> DETENCION_C : [etapa == 2]
        DETENCION_C -> DESCENSO_C : [etapa == 3]
        MOVIMIENTO.AUTOMATICO.IZAJE.INICIO -> DESCENSO_C [order 3] : [etapa == 3 && cargando]
        MOVIMIENTO.AUTOMATICO.IZAJE.INICIO -> DETENCION_C [order 2] : [(etapa == 2 || etapa == 4) && cargando]
        MOVIMIENTO.AUTOMATICO.IZAJE.INICIO -> ASCENSO_C [order 1] : [etapa ==1 && cargando]
        (default) -> MOVIMIENTO.AUTOMATICO.IZAJE.INICIO
        MOVIMIENTO.AUTOMATICO.IZAJE.INICIO -> DESCENSO_D [order 5] : [etapa == 2 && ~cargando]
        MOVIMIENTO.AUTOMATICO.IZAJE.INICIO -> ASCENSO_D [order 6] : [etapa == 4 && ~cargando]
        MOVIMIENTO.AUTOMATICO.IZAJE.INICIO -> DETENCION_D [order 4] : [(etapa == 1 || etapa == 3) && ~cargando]
        ASCENSO_D -> DETENCION_D : [etapa == 3]
        DETENCION_D -> DESCENSO_D : [etapa == 2]
    (default) -> MANUAL
    MANUAL -> AUTOMATICO : [Auto && etapa ~= 0 && etapa ~= 5]
    AUTOMATICO -> MANUAL : [~Auto || etapa == 5 || etapa == 0]
  state TRAYECTORIA [parallel]
    during:
    v_i_max = vMaxIzaje(m_l);
    [h, l] = corregirTrayectoria(H, L, cargando, cargaM, vx, vy);
    settings: executionOrder=1
    state ETAPA2
      entry:
      etapa = 2;
    state ETAPA3
      entry:
      etapa = 3;
    state ETAPA1
      entry:
      etapa = 1;
    state ETAPA4
      entry:
      etapa = 4;
    state HOMING_C
      during: etapa = 6;
      if (x < l(2) - 1)
      C_dx_c = 0.05 * v_c_max;
      elseif (x > l(2) + 1)
      C_dx_c = -0.05 * v_c_max;
      end
      if (y < h(2) - 1)
      C_dx_i = -0.05 * v_i_max;
      elseif (x > l(2) + 1)
      C_dx_i = 0.05 * v_i_max;
      end
    state HOMING_D
      during: etapa = 6;
      if (x < l(5) - 1)
      C_dx_c = 0.05 * v_c_max;
      elseif (x > l(5) + 1)
      C_dx_c = -0.05 * v_c_max;
      end
      if (y < h(5) - 1)
      C_dx_i = -0.05 * v_i_max;
      elseif (x > l(5) + 1)
      C_dx_i = 0.05 * v_i_max;
      end
    state ETAPA0
      entry:
      etapa = 0;
    state INI
    state ETAPA5
      entry:
      etapa = 5;
    ETAPA1 -> ETAPA2 [order 1] : [cargando && y >= h(3) && x >= l(3)]
    ETAPA3 -> ETAPA4 [order 1] : [cargando && y <= h(5) && x >= l(5)]
    ETAPA2 -> ETAPA3 [order 1] : [cargando && y >= h(4) && x >= l(4)]
    ETAPA3 -> ETAPA2 [order 2] : [~cargando && y >= h(3) && x <= l(3)]
    ETAPA4 -> ETAPA3 [order 2] : [~cargando && y >= h(4) && x <= l(4)]
    ETAPA2 -> ETAPA1 [order 2] : [~cargando && y <= h(2) && x <= l(2)]
    ETAPA2 -> INI [order 3] : [~Auto]
    ETAPA3 -> INI [order 3] : [~Auto]
    HOMING_C -> ETAPA1 [order 1] : [vx >= -0.2 && vx <=0.2 && vy >= -0.2 && vy <= 0.2 && x >= l(2) - 1 && x <= l(2) + 1 && y >= h(2) - 1 && y <= h(2) + 1]
    ETAPA1 -> INI [order 3] : [~Auto]
    ETAPA4 -> INI [order 3] : [~Auto]
    ETAPA4 -> ETAPA5 [order 1] : [cargando && y <= h(6)]
    ETAPA1 -> ETAPA0 [order 2] : [~cargando && y <= h(1)]
    HOMING_D -> ETAPA4 [order 1] : [vx >= -0.2 && vx <=0.2 && vy >= -0.2 && vy <= 0.2 && x >= l(5) - 1 && x <= l(5) + 1 && y >= h(5) - 1 && y <= h(5) + 1]
    HOMING_C -> INI [order 2] : [~Auto]
    HOMING_D -> INI [order 2] : [~Auto]
    ETAPA0 -> HOMING_C [order 1] : [cargando && y >= h(2) && x >= l(2)]
    ETAPA5 -> HOMING_D [order 1] : [~cargando && y >= h(5) && x <= l(5)]
    ETAPA0 -> INI [order 2] : [~Auto]
    ETAPA5 -> INI [order 2] : [~Auto]
    INI -> ETAPA0 [order 1] : [cargando]
    INI -> ETAPA5 [order 2] : [~cargando]
    (default) -> INI
  data: m function_input; vMax function_output; H_ function_input; L_ function_input; H_1 function_output; L_1 function_output; carga_op function_input; carga_masa function_input; v_x function_input; v_y function_input; m function_input; vMax function_output; m_l input; C_dx_c output; C_dx_i output; Comando_i input; Comando_c input; v_c_max parameter; v_i_max local; Auto input; etapa local; h local size=6; l local size=6; x input; y input; cargando input; vx input; vy input; modo_ output; H parameter; L parameter; cargaM input
  function vMax = vMaxIzaje(m):
    | function vMax = vMaxIzaje(m)
    |     g = 9.8;
    |     if (m <= 32500)
    |         vMax = 956150 / (32500 * g);
    |     elseif (m <= 65000)
    |         vMax = 956150 / (m * g);
    |     else
    |         vMax = 0; %Por seguridad, si la masa total excede los 65000 kg no elevarla.
    |     end
    | end
  function [H_1, L_1]  = corregirTrayectoria (H_, L_, carga_op, carga_masa, v_x, v_y):
    | function [H_1, L_1]  = corregirTrayectoria (H_, L_, carga_op, carga_masa, v_x, v_y)    
    |     H_1 = H_;
    |     L_1 = L_;
    |     % Corrección inercia
    |     if (carga_masa)
    |         if (carga_op)
    |             H_1(2) = H_(2) + 2.0;
    |             H_1(3) = H_(3) + v_y * 1.1;
    |             L_1(3) = L_(3) - v_x * 1.1;
    |             L_1(4) = L_(4) - v_x * 2.6;
    |             H_1(6) = H_(6) + v_y * 2.8;
    |         else
    |             H_1(5) = H_(5) - 7;
    |             L_1(4) = L_(4) - v_x * 1.0;
    |             H_1(4) = H_(4) + v_y * 1.0;
    |             L_1(3) = L_(3) + v_x * 2.1;
    |             H_1(1) = H_(1) + v_y + 1.9;
    |         end
    |     else
    |         if (carga_op)
    |             H_1(2) = H_(2) - 10;
    |             H_1(3) = H_(3) + v_y * 1.8;
    |             L_1(3) = L_(3) - v_x * 1.8;
    |             L_1(4) = L_(4) - v_x * 2.6;
    |             H_1(6) = H_(6) + v_y * 2.8;
    |         else
    |             H_1(5) = H_(5) - 5;
    |             L_1(4) = L_(4) - v_x * 1.2;
    |             H_1(4) = H_(4) + v_y * 1.2;
    |             L_1(3) = L_(3) + v_x * 2.0;
    |             H_1(1) = H_(1) + v_y + 1.5;
    |         end
    |     end
    | end
  function vMax = vMaxIzaje(m):
    | function vMax = vMaxIzaje(m)
    |     g = 9.8;
    |     if (m <= 32500)
    |         vMax = 956150 / (32500 * g);
    |     elseif (m <= 65000)
    |         vMax = 956150 / (m * g);
    |     else
    |         vMax = 0; %Por seguridad, si la masa total excede los 65000 kg no elevarla.
    |     end
    | end

== stateflow chart Sistema_completo/Graficas ==
  state Grafico
    entry:
    contador=0;
    pl_cable=plot([xt xl],[45 yl],'Color','k');
    pl_carro=rectangle('Position',[xt-2, 45, 4, 2 ],'FaceColor','r');
    pl_spreder=rectangle('Position',[xl-0.6, yl+1.3,1.2,.2],'FaceColor','k');
    pl_trayectoria=plot(xl,yl,'om','MarkerSize',3,'MarkerFaceColor','m');
    pl_carga=rectangle('Position',[xl-1.2,yl-1.3,2.4,2.6],'FaceColor','b');
    during:
    plot_dinamico();
    plot_indicadores();
  (default) -> Grafico
  data: xl input; xt input; yl input; pl_cable local; pl_carga local; pl_carro local; pl_spreder local; cargado input; alarma input; automatico input; balanceo input; contador local; pl_trayectoria local
  function plot_dinamico:
    | function plot_dinamico()
    | contador=contador+1;   
    | 
    | if contador==7
    |     
    |     contador=0;
    |     %carro
    |     set(pl_carro,'visible','off');
    |     pl_carro=rectangle('Position',[xt-2, 45, 4, 2 ],'FaceColor','r');
    |     
    |     %cable
    |     set(pl_cable,'visible', 'off');
    |     pl_cable=plot([xt xl],[45 yl],'Color','k');
    |     
    |    %spreder
    |     set(pl_spreder, 'visible','off');
    |     pl_spreder=rectangle('Position',[xl-0.6, yl+1.3,1.2,.2],'FaceColor','k');
    |     
    |     
    |     %trayectoria
    |     pl_trayectoria=plot(xl,yl,'om','MarkerSize',3,'MarkerFaceColor','m');
    |     
    |     %carga
    |     if cargado==0
    |         set(pl_carga,'visible','off');
    |     end
    |     
    |     if cargado==1
    |         set(pl_carga,'visible','off');
    |         pl_carga=rectangle('Position',[xl-1.2,yl-1.3,2.4,2.6],'FaceColor','b');
    |     end
    |     
    |     
    |     
    |  end
    |     
    |     
    | end
  function plot_indicadores:
    | function plot_indicadores
    | 
    | if balanceo==1
    |      plot(-3,-18.5,'og','MarkerSize',10,'MarkerFaceColor','g');
    | end
    | if balanceo==0
    |      plot(-3,-18.5,'or','MarkerSize',10,'MarkerFaceColor','r');
    | end
    | 
    | if alarma==1
    |      plot(-3,-13.5,'og','MarkerSize',10,'MarkerFaceColor','g');
    | end
    | if alarma==0
    |      plot(-3,-13.5,'or','MarkerSize',10,'MarkerFaceColor','r');
    | end
    | 
    | if automatico==1
    |      plot(-3,-8.5,'og','MarkerSize',10,'MarkerFaceColor','g');
    | end
    | if automatico==0
    |      plot(-3,-8.5,'or','MarkerSize',10,'MarkerFaceColor','r');
    | end
    | 
    | if cargado==1
    |      plot(-3,-3.5,'og','MarkerSize',10,'MarkerFaceColor','g');
    | end
    | if cargado==0
    |      plot(-3,-3.5,'or','MarkerSize',10,'MarkerFaceColor','r');
    | end
    | 
    | 
    | end

== matlab function Sistema_completo/ Planta/Subsistema Carga/MATLAB Function ==
  data: xl input; yc0 output; X_contenedores input; Y_contenedores input; charged input
function yc0 = getYc0x(xl, X_contenedores, Y_contenedores, charged)
yc0 = 2.6;
aux = 0;
indice = 1;
if(xl <= 0)
    yc0 = 0;
    
elseif (xl >= 50)
    yc0 = 0;
    
elseif (xl > 0)
   for i=1:length(X_contenedores)
       % xl hasta centro columna
       x_comp = xl-X_contenedores(i);
        if(x_comp>= -2.5 && x_comp<0)
            if (i ~= 1 && Y_contenedores(i-1)>=Y_contenedores(i))
                indice = i-1;
            else
                indice = i;
            end
        elseif(x_comp == 0)
            indice = i;
        elseif(x_comp<= 2.5 && x_comp>0)
            if (i ~= length(X_contenedores) && Y_contenedores(i+1)>=Y_contenedores(i))
                indice = i+1;
            else
                indice = i;
            end
        end 
    end
    yc0=Y_contenedores(indice);
end

if(charged == 1)
    yc0 = yc0 + 2.5/2;
end
    
end

== matlab function Sistema_completo/MATLAB Function ==
  data: L output; R output; cuadrado output; o output; x output; triangulo output; u input; Select output; Start output
function [L, R, cuadrado, o, x, triangulo, Select, Start] = buttonMap(u)
    x = double(bitand(u, 1));
    
    u = bitshift(u, -1);
    o = double(bitand(u, 1));
    
    u = bitshift(u, -1);
    cuadrado = double(bitand(u, 1));
    
    u = bitshift(u, -1);
    triangulo = double(bitand(u, 1));
    
    u = bitshift(u, -1);
    L = double(bitand(u, 1));
    
    u = bitshift(u, -1);
    R = double(not(bitand(u, 1)));
    
    u = bitshift(u, -1);
    Select = double(bitand(u, 1));
    
    u = bitshift(u, -1);
    Start = double(bitand(u, 1));
end

== stateflow chart Sistema_completo/Autómata Nivel 0/Chart1 ==
  state WATCHDOG [parallel]
    settings: executionOrder=2
    state REINICIO
      entry:
      contador = 0;
    state BOTTOM
      during:
      contador = contador + 1;
    state TOP
      during:
      contador = contador + 1;
    state EMERGENCIA
      entry:
      dl_i = 0;
      dx_c = 0;
      alerta = 1;
      exit:
      alerta = 0;
    (default) -> REINICIO
    EMERGENCIA -> REINICIO : [reset == 1]
    TOP -> REINICIO [order 1] : [WD == 0]
    REINICIO -> BOTTOM
    BOTTOM -> EMERGENCIA [order 2] : [contador > 5000]
    BOTTOM -> TOP [order 1] : [WD == 1]
    TOP -> EMERGENCIA [order 2] : [contador > 5000]
  state CONTROL [parallel]
    settings: executionOrder=1
    state OK
      entry:
      alerta = 0;
    state PARADA
      entry:
      dl_i = 0;
      dx_c = 0;
      alerta = 1
    state FIN_CARRERA
      state Fin_carrera_c [parallel]
        entry:
        if (fin_D)
        dx_c = -4;
        elseif (fin_I)
        dx_c = 4;
        end
        alerta = 1;
        during:
        if (fin_D || fin_I)
        dx_c = 0;
        if (~(fin_A || fin_U))
        dl_i = C_dx_i;
        end
        end
        settings: executionOrder=1
      state Fin_carrera_i [parallel]
        entry:
        if (fin_A)
        dl_i = -4;
        elseif (fin_U)
        dl_i = 4;
        end
        alerta = 1;
        during:
        if (fin_A || fin_U)
        dl_i = 0;
        if (~(fin_D || fin_I))
        dx_c = C_dx_c;
        end
        end
        settings: executionOrder=2
    state SENSORES
      entry:
      alerta = 1;
      dl_i = 0;
      dx_c = 0;
    state EXCESO
      entry:
      alerta = 1;
      control_velocidad;
    (default) -> OK
    PARADA -> OK : [stop == 0 && reset == 1]
    SENSORES -> OK : [sensores == 1 && reset == 1]
    OK -> PARADA [order 2] : [stop == 1]
    OK -> SENSORES [order 5] : [sensores == 0]
    EXCESO -> OK : [estable == 1]
    OK -> EXCESO [order 4] : [C_dx_i > lim_vh]
    FIN_CARRERA -> OK : [~fin_A && ~fin_U && ~fin_I && ~fin_D]
    OK -> FIN_CARRERA [order 1] : [fin_A || fin_U || fin_D || fin_I]
    OK -> EXCESO [order 3] : [C_dx_c > lim_vt]
  data: dx_c output; dl_i output; contador local =0; C_dx_c input; C_dx_i input; estable local; fin_A input; fin_D input; fin_I input; fin_U input; lim_vt local =10; lim_vh local =10; sensores input; stop input; alerta output; WD input; reset input
  function control_velocidad:
    | function control_velocidad
    | vt=C_dx_c;
    | vh=C_dx_i;
    | 
    | 
    |     if C_dx_c>=lim_vt
    |        while vh>=lim_vt*.8
    |            vt=vt*.95;
    |        end
    |     end
    |        estable=1;
    |     if C_dx_i>=lim_vh
    |        while vh>=lim_vh*.8
    |            vh=vh*.95;
    |        end
    |        estable=1;
    |     end
    |     end

== matlab function Sistema_completo/ Planta/Longitud y Ángulo Cable ==
  data: Theta output; l output; x_c input; x_l input; y_l input; y_t0 input
function [Theta, l]= longitudAnguloCable(x_c, x_l, y_l, y_t0)
    a = x_l - x_c;
    b = y_t0 - y_l;
    l = sqrt(a^2 + b^2);
    Theta = atan2(a, b);
end
